simulink model "TRN"  (R2022a)
settings: Solver=FixedStepAuto  StartTime=0.0  StopTime=300  FixedStep=0.04  RelTol=1e-3
PreLoadFcn:
  | load('BusStructureTRNsensor.mat');
  | addpath('C:/MAP');
InitFcn:
  | %load TRNDataBusPILS.mat
  | %addpath(genpath(cd))
  | 
  | load('TPF_WHOLESIM_INPUT_SCENARIOS_AGCAS_N35_10E127_70.mat');
  | 
  | % Add DataBus Path
  | addpath(',,/');
  | addpath('../MAP/');
  | addpath('../MAP/MAP_DB');
  | addpath('../MAP/DVOF');
  | addpath(genpath(cd));
  | load('BusStructureTRN.mat');
undefined symbols (not defined in the file or in its folder): Altitude_INS, INSDataNotValid, Latitude_INS, Longitude_INS, TRN, TRNlib
libraries: simulink_extras x26, aerolibconvert2 x14, sharedtransform x3, dspstat3 x2
(part 1 of 3)
settings Model: Creator=HSU  LastModifiedBy=20225
settings OptimizationCC: DefaultParameterBehavior=Inlined  UseDivisionForNetSlopeComputation=on  GainParamInheritBuiltInType=on  UseFloatMulNetSlope=on  PassReuseOutputArgsAs=Individual arguments  ZeroExternalMemoryAtStartup=off  ZeroInternalMemoryAtStartup=off  OptimizeBlockOrder=speed  DifferentSizesBufferReuse=on  EfficientTunableParamExpr=on
settings DebuggingCC: ParameterTunabilityLossMsg=error  UnconnectedInputMsg=warning  UnconnectedOutputMsg=warning  UnconnectedLineMsg=warning  SFUnexpectedBacktrackingDiag=warning  SFNoUnconditionalDefaultTransitionDiag=warning
settings HardwareCC: ProdBitPerPointer=32  ProdBitPerSizeT=32  ProdBitPerPtrDiffT=32  ProdLargestAtomicInteger=Long  ProdLargestAtomicFloat=Double  ProdEndianess=BigEndian  ProdWordSize=32  ProdHWDeviceType=Freescale->MPC83xx
settings ModelReferenceCC: ModelReferenceNumInstancesAllowed=Single
settings SFSimCC: SimUserLibraries=MAPd.lib WS2_32.LIB  MATLABDynamicMemAlloc=off
settings SFSimCC: SimCustomHeaderCode=|
  | #include "MAP.h"
  | #include "MAPDATA.h"
  | #include "DVOF.h"
  | #include "userDefined.h"
settings SFSimCC: SimUserSources=|
  | MAP.c
  | DVOF.c
  | userDefined.c
settings RTWCC: SystemTargetFile=ert.tlc  GenCodeOnly=on  TemplateMakefile=ert_default_tmf  GenerateReport=on  RTWUseSimCustomCode=on  CustomLibrary=MAPd.lib WS2_32.LIB  BuildConfiguration=Faster Runs  LaunchReport=on  DLArmComputeVersion=19.05
settings RTWCC: CustomHeaderCode=|
  | #include "MAP.h"
  | #include "MAPDATA.h"
  | #include "DVOF.h"
  | #include "userDefined.h"
settings RTWCC: CustomSource=|
  | MAP.c
  | DVOF.c
  | userDefined.c
settings CodeAppCC: ForceParamTrailComments=on  IgnoreCustomStorageClasses=off  OperatorAnnotations=on  SimulinkDataObjDesc=on  SFDataObjDesc=on  MATLABFcnDesc=on  InsertBlockDesc=on  StateflowObjectComments=on  MATLABSourceComments=on  EnableCustomComments=on  ReqsInCode=on
settings ERTTargetCC: TargetLangStandard=C99 (ISO)  UtilityFuncGeneration=Shared location  GenerateSampleERTMain=on  SuppressErrorStatus=on  SupportAbsoluteTime=off  SupportNonFinite=off  SupportComplex=off  ParenthesesLevel=Standards  CastingMode=Standards  InlinedParameterPlacement=NonHierarchical  ERTCustomFileTemplate=example_file_process.tlc  PreserveIfCondition=on  ConvertIfToSwitch=off  EnableSignedLeftShifts=off  EnableSignedRightShifts=off

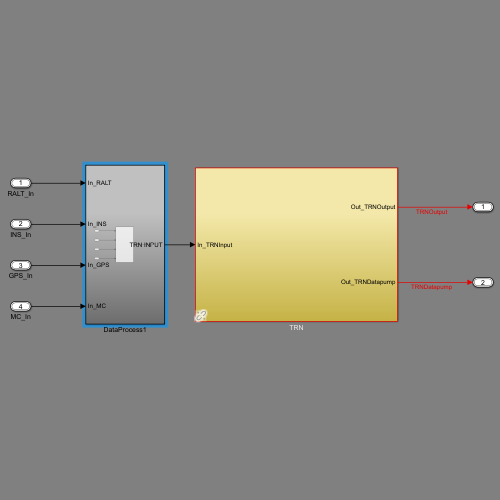
[thumbnail: Simulink's stored preview of the top-level diagram]
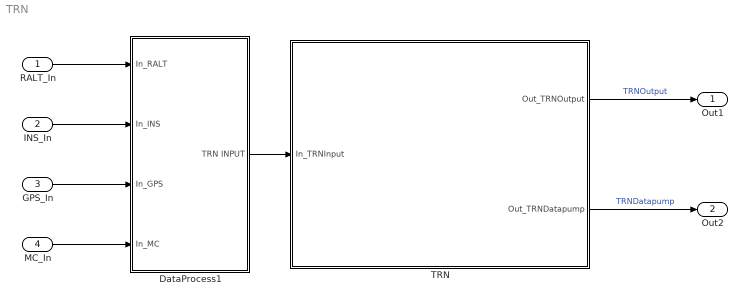
== system TRN ==
  RALT_In : Inport  OutDataTypeStr=Bus: BUS_SENSOR_RALT
  INS_In : Inport  Port=2  OutDataTypeStr=Bus: BUS_SENSOR_INS
  GPS_In : Inport  Port=3  OutDataTypeStr=Bus: BUS_SENSOR_GPS
  MC_In : Inport  Port=4  OutDataTypeStr=Bus: TRN_MC
  DataProcess1 : Subsystem
  TRN : Subsystem  AncestorBlock=TRNlib/TRN
  Out1 : Outport  OutDataTypeStr=Bus: TRNOutput  VectorParamsAs1DForOutWhenUnconnected=off
  Out2 : Outport  Port=2  OutDataTypeStr=Bus: TRNDatapump  VectorParamsAs1DForOutWhenUnconnected=off
  wires:
  TRN/2(Out_TRNDatapump) -> Out2/1  "TRNDatapump"
  TRN/1(Out_TRNOutput) -> Out1/1  "TRNOutput"
  RALT_In/1 -> DataProcess1/1(In_RALT)
  INS_In/1 -> DataProcess1/2(In_INS)
  GPS_In/1 -> DataProcess1/3(In_GPS)
  DataProcess1/1(TRN INPUT) -> TRN/1(In_TRNInput)
  MC_In/1 -> DataProcess1/4(In_MC)

== system TRN/DataProcess1 ==
  In_RALT : Inport
  In_INS : Inport  Port=2
  In_GPS : Inport  Port=3
  In_MC : Inport  Port=4
  Subsystem3 : Subsystem
  TRN INPUT : Outport
  wires:
  In_GPS/1 -> Subsystem3/3(In_GPS)
  In_MC/1 -> Subsystem3/4(In_MC)
  Subsystem3/1(TRN INPUT) -> TRN INPUT/1
  In_RALT/1 -> Subsystem3/1(In_RALT)
  In_INS/1 -> Subsystem3/2(In_INS)

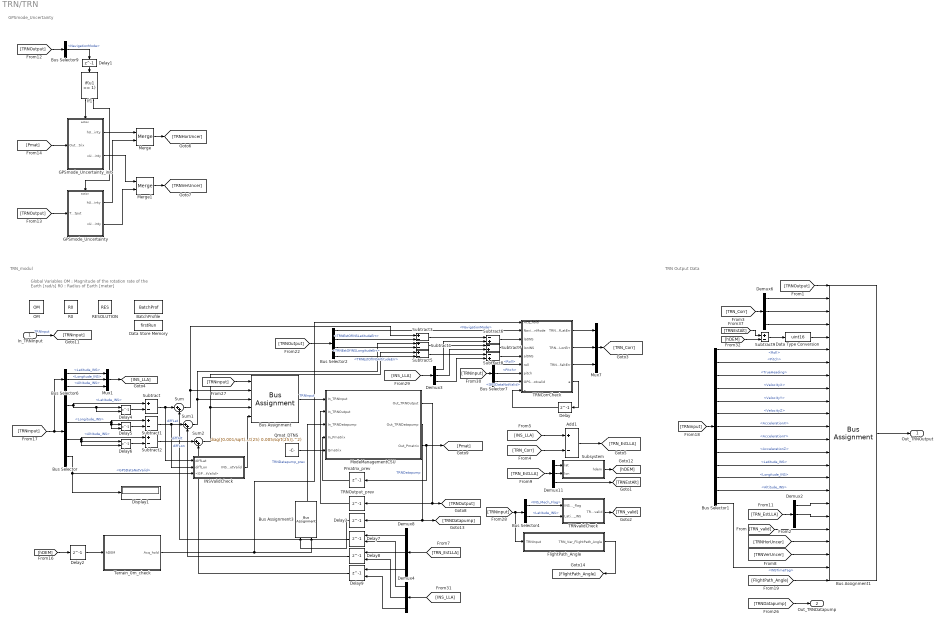
== system TRN/TRN ==
  note: Global Variables
      | OM : Magnitude of the rotation rate of the Earth [rad/s]
      | R0 : Radius of Earth [meter]
  note: GPSmode_Uncertainty
  note: TRN Output Data
  note: TRN_modul
  In_TRNInput : Inport  OutDataTypeStr=Bus: TRNInput
  Add1 : Sum  Inputs=+-
  BatchProfile : DataStoreMemory  DataStoreName=BatchProf  ReadBeforeWriteMsg=warning  WriteAfterWriteMsg=warning  WriteAfterReadMsg=warning  ShowAdditionalParam=off  OutDataTypeStr=double  Dimensions=84200
  Bus Assignment : BusAssignment  AssignedSignals=Latitude_INS,Longitude_INS,Altitude_INS,INSDataNotValid
  Bus Assignment1 : BusAssignment  AssignedSignals=TRNEstOfINSLatitudeErr,TRNEstOfINSLongitudeErr,TRNEstOfINSAltitudeErr,TRNEstHeightAGL,TRN_Roll,TRN_Pitch,TRN_Yaw,TRN_VelocityX,TRN_VelocityY,TRN_VelocityZ,TRN_AccelerationX,TRN_AccelerationY,TRN_AccelerationZ,Latitude_INS,Longitude_INS,Altitude_INS,TRNEstOfLatitude,TRNEstOfLongitude,TRN_valid,TRNHorUncertainty,TRNVerticalUncertainty,TRNTimeTag,TRN_Ver_FlightPath_Angle
  Bus Assignment3 : BusAssignment  AssignedSignals=Acq_hold
  Bus Selector : BusSelector  OutputSignals=Latitude_INS,Longitude_INS,Altitude_INS,GPSDataNotValid
  Bus Selector1 : BusSelector  OutputSignals=Roll,Pitch,TrueHeading,VelocityX,VelocityY,VelocityZ,AccelerationX,AccelerationY,AccelerationZ,Latitude_INS,Longitude_INS,Altitude_INS,INSTimeTag
  Bus Selector2 : BusSelector  OutputSignals=NavigationMode,TRNEstOfINSLatitudeErr,TRNEstOfINSLongitudeErr,TRNEstOfINSAltitudeErr
  Bus Selector4 : BusSelector  OutputSignals=INS_Mech_Flag,Latitude_INS
  Bus Selector6 : BusSelector  OutputSignals=Latitude_INS,Longitude_INS,Altitude_INS
  Bus Selector7 : BusSelector  OutputSignals=Roll,Pitch,GPSDataNotValid
  Bus Selector9 : BusSelector  OutputSignals=NavigationMode
  Data Store Memory : DataStoreMemory  DataStoreName=firstRun  ReadBeforeWriteMsg=warning  WriteAfterWriteMsg=warning  WriteAfterReadMsg=warning  InitialValue=logical(1)  VectorParams1D=off  ShowAdditionalParam=off  OutDataTypeStr=boolean
      settings: LockScale=on
  Data Type Conversion : DataTypeConversion  OutDataTypeStr=uint16  RndMeth=Nearest  SaturateOnIntegerOverflow=off
  Delay : Delay  DelayLength=1
  Delay1 : Delay  DelayLength=1  InitialCondition=1
  Delay2 : Delay  DelayLength=1
  Delay3 : Delay  DelayLength=1  InitialCondition=0
  Delay4 : Delay  DelayLength=1  InitialConditionSource=Input port  InitialCondition=35.2*pi/180
      settings: InputPortMap=u0,p4
  Delay5 : Delay  DelayLength=1  InitialConditionSource=Input port  InitialCondition=35.2*pi/180
      settings: InputPortMap=u0,p4
  Delay6 : Delay  DelayLength=1  InitialConditionSource=Input port  InitialCondition=35.2*pi/180
      settings: InputPortMap=u0,p4
  Delay7 : Delay  DelayLength=1  InitialConditionSource=Input port  InitialCondition=0
      settings: InputPortMap=u0,p4
  Delay8 : Delay  DelayLength=1  InitialConditionSource=Input port  InitialCondition=0
      settings: InputPortMap=u0,p4
  Delay9 : Delay  DelayLength=1  InitialConditionSource=Input port  InitialCondition=0
      settings: InputPortMap=u0,p4
  Demux{2..4,6,8,11} (6 alike) : Demux  Outputs=3
  Display1 : Display
  FlightPath_Angle : Subsystem  TreatAsAtomicUnit=on
  GPSmode_Uncertainty : Subsystem  TreatAsAtomicUnit=on
  GPSmode_Uncertainty_init : Subsystem  TreatAsAtomicUnit=on
  INSValidCheck : Subsystem
  If1 : If  IfExpression=u1 == 1
  Merge : Merge
  Merge1 : Merge
  ModeManagementCSU : Stateflow chart  TreatAsAtomicUnit=on
  Mux1 : Mux  Inputs=3
  Mux7 : Mux  Inputs=3
  OM : DataStoreMemory  DataStoreName=OM  ReadBeforeWriteMsg=warning  WriteAfterWriteMsg=warning  WriteAfterReadMsg=warning  InitialValue=7.27e-5  ShowAdditionalParam=off
  Pmatrix_prev : Delay  DelayLength=1  InitialCondition="diag([0 0 0 0 0 0  10/6378000 10/6378000 13.3 0.0 0.0 0.0 0.00014 0.00014 0.00014 ].^2);"
  Qmat_DTNS : Constant  Value=diag([0.001/sqrt(25) 0.001/sqrt(25) 0.001/sqrt(25) 0.005/sqrt(25) 0.005/sqrt(25) 0.005/sqrt(25)].^2)
  R0 : DataStoreMemory  DataStoreName=R0  ReadBeforeWriteMsg=warning  WriteAfterWriteMsg=warning  WriteAfterReadMsg=warning  InitialValue=6378000  ShowAdditionalParam=off
  RESOLUTION : DataStoreMemory  DataStoreName=RES  ReadBeforeWriteMsg=warning  WriteAfterWriteMsg=warning  WriteAfterReadMsg=warning  InitialValue=3 * 0.000277777777777777 * 0.0174532925199433  ShowAdditionalParam=off  OutDataTypeStr=double
  Subsystem : Subsystem
  Subtract{,1..5,9} (7 alike) : Sum  Inputs=+-
  Subtract6 : Sum  Inputs=-+
  Subtract7 : Sum  Inputs=-+
  Subtract8 : Sum  Inputs=-+
  Sum : Sum  Inputs=|++
  Sum1 : Sum  Inputs=|++
  Sum2 : Sum  Inputs=|++
  TRNCorrCheck : MATLAB Function  TreatAsAtomicUnit=on
  TRNOutput_prev : Delay  DelayLength=1  InitialCondition=struct('NavigationMode', false);
  TRNvalidCheck : MATLAB Function  TreatAsAtomicUnit=on
  Terrain_0m_check : MATLAB Function  TreatAsAtomicUnit=on
  Out_TRNOutput : Outport  OutDataTypeStr=Bus: TRNOutput  VectorParamsAs1DForOutWhenUnconnected=off
  Out_TRNDatapump : Outport  Port=2  OutDataTypeStr=Bus: TRNDatapump  VectorParamsAs1DForOutWhenUnconnected=off
  wires:
  Bus Selector2/3 -> Subtract4/2  "<TRNEstOfINSLongitudeErr>"
  Bus Selector2/2 -> Subtract3/2  "<TRNEstOfINSLatitudeErr>"
  Subsystem/1(hdem) -> [hDEM]
  Bus Selector4/1 -> TRNvalidCheck/1(INS_Mech_flag)  "<INS_Mech_Flag>"
  Bus Selector4/2 -> TRNvalidCheck/2(Latitude_INS)  "<Latitude_INS>"
  [TRN_valid] -> Bus Assignment1/20
  TRNvalidCheck/1(TRN_valid) -> [TRN_valid]
  Bus Assignment/1 -> ModeManagementCSU/1(In_TRNInput)  "TRNInput"
  Bus Selector/2 -> Subtract1/1, Delay5/1, Delay5/2  "<Longitude_INS>"
  Bus Selector1/3 -> Bus Assignment1/8  "<TrueHeading>"
  Bus Selector1/12 -> Bus Assignment1/17  "<Altitude_INS>"
  Bus Selector1/11 -> Bus Assignment1/16  "<Longitude_INS>"
  Bus Selector1/10 -> Bus Assignment1/15  "<Latitude_INS>"
  Bus Selector1/9 -> Bus Assignment1/14  "<AccelerationZ>"
  Bus Selector1/8 -> Bus Assignment1/13  "<AccelerationY>"
  Bus Selector1/7 -> Bus Assignment1/12  "<AccelerationX>"
  Bus Selector1/6 -> Bus Assignment1/11  "<VelocityZ>"
  Bus Selector1/5 -> Bus Assignment1/10  "<VelocityY>"
  Bus Selector1/4 -> Bus Assignment1/9  "<VelocityX>"
  Bus Selector1/2 -> Bus Assignment1/7  "<Pitch>"
  Bus Selector1/1 -> Bus Assignment1/6  "<Roll>"
  In_TRNInput/1 -> [TRNinput]  "TRNInput"
  ModeManagementCSU/1(Out_TRNOutput) -> TRNOutput_prev/1, [TRNOutput]
  ModeManagementCSU/2(Out_TRNDatapump) -> Delay3/1, [TRNDatapump]  "TRNDatapump"
  Pmatrix_prev/1 -> ModeManagementCSU/4(In_Pmatrix)
  TRNOutput_prev/1 -> ModeManagementCSU/2(In_TRNOutput)
  Delay3/1 -> Bus Assignment3/1
  Bus Selector/3 -> Subtract2/1, Delay6/2, Delay6/1  "<Altitude_INS>"
  Bus Selector/1 -> Subtract/1, Delay4/1, Delay4/2  "<Latitude_INS>"
  Delay4/1 -> Subtract/2
  Delay5/1 -> Subtract1/2
  Delay6/1 -> Subtract2/2
  Sum/1 -> Subtract3/1, Bus Assignment/2
  Sum1/1 -> Subtract4/1, Bus Assignment/3
  Sum2/1 -> Subtract5/1, Bus Assignment/4
  Subtract/1 -> Sum/1, INSValidCheck/1(diffLat)  "diffLat"
  Subtract1/1 -> INSValidCheck/2(diffLon), Sum1/1  "diffLon"
  Subtract4/1 -> Subtract7/1
  Subtract2/1 -> Sum2/1  "diffAlt"
  Delay7/1 -> Sum/2
  Delay8/1 -> Sum1/2
  Delay9/1 -> Sum2/2
  Bus Assignment1/1 -> Out_TRNOutput/1
  Subtract9/1 -> Data Type Conversion/1
  Data Type Conversion/1 -> Bus Assignment1/5
  Subtract6/1 -> TRNCorrCheck/3(latINS)
  Subtract7/1 -> TRNCorrCheck/4(lonINS)
  Subtract8/1 -> TRNCorrCheck/5(altINS)
  TRNCorrCheck/3(TRNEstOfaltErr) -> Mux7/3
  [TRN_Corr] -> Demux6/1
  Demux6/1 -> Bus Assignment1/2
  Demux6/2 -> Bus Assignment1/3
  Demux6/3 -> Bus Assignment1/4
  TRNCorrCheck/1(TRNEstOfLatErr) -> Mux7/1
  TRNCorrCheck/2(TRNEstOfLonErr) -> Mux7/2
  Subtract5/1 -> Subtract8/1
  Subtract3/1 -> Subtract6/1
  [TRN_EstLLA] -> Demux8/1
  Demux8/1 -> Delay7/1
  Demux8/2 -> Delay8/1
  Demux8/3 -> Delay9/1
  Mux1/1 -> [INS_LLA]
  Bus Selector6/2 -> Mux1/2  "<Longitude_INS>"
  Bus Selector6/3 -> Mux1/3  "<Altitude_INS>"
  [INS_LLA] -> Add1/1
  [TRN_Corr] -> Add1/2
  Add1/1 -> [TRN_EstLLA]
  Demux11/1 -> Subsystem/1(lat)
  Demux11/2 -> Subsystem/2(lon)
  TRNCorrCheck/4(a) -> Delay/1
  Delay/1 -> TRNCorrCheck/9("a ")
  [TRN_EstLLA] -> Demux11/1
  Qmat_DTNS/1 -> ModeManagementCSU/5(Qmatrix)
  ModeManagementCSU/3(Out_Pmatrix) -> Pmatrix_prev/1, [Pmat]
  INSValidCheck/1(INSDataNotValid) -> Bus Assignment/5
  Bus Selector/4 -> Display1/1, INSValidCheck/3(<GPSDataNotValid>)  "<GPSDataNotValid>"
  Mux7/1 -> [TRN_Corr]
  If1/1 -> GPSmode_Uncertainty_init/Action
  If1/2 -> GPSmode_Uncertainty/Action
  GPSmode_Uncertainty_init/1(hUncertainty) -> Merge/1
  GPSmode_Uncertainty/1(hUncertainty) -> Merge/2
  GPSmode_Uncertainty_init/2(vUncertainty) -> Merge1/1
  GPSmode_Uncertainty/2(vUncertainty) -> Merge1/2
  Bus Selector9/1 -> Delay1/1  "<NavigationMode>"
  Merge/1 -> [TRNHorUncer]
  Merge1/1 -> [TRNVerUncer]
  [TRNHorUncer] -> Bus Assignment1/21
  [TRNVerUncer] -> Bus Assignment1/22
  Demux2/1 -> Bus Assignment1/18
  Demux2/2 -> Bus Assignment1/19
  [TRN_EstLLA] -> Demux2/1
  [TRNOutput] -> Bus Selector9/1
  [TRNOutput] -> GPSmode_Uncertainty/1(TRNOutput)
  [Pmat] -> GPSmode_Uncertainty_init/1(Out_Pmatrix)
  [TRNinput] -> Bus Selector6/1, Bus Selector/1
  [TRNinput] -> Bus Selector1/1
  [TRNDatapump] -> Out_TRNDatapump/1
  [TRNinput] -> Bus Assignment/1
  Delay1/1 -> If1/1
  [TRNOutput] -> Bus Assignment1/1
  Bus Selector2/4 -> Subtract5/2  "<TRNEstOfINSAltitudeErr>"
  [TRNOutput] -> Bus Selector2/1
  [INS_LLA] -> Demux3/1
  Demux3/1 -> Subtract6/2
  Demux3/2 -> Subtract7/2
  Demux3/3 -> Subtract8/2
  [TRNinput] -> Bus Selector7/1
  Bus Selector7/1 -> TRNCorrCheck/6(roll)  "<Roll>"
  Bus Selector7/2 -> TRNCorrCheck/7(pitch)  "<Pitch>"
  Bus Selector6/1 -> Mux1/1  "<Latitude_INS>"
  [INS_LLA] -> Demux4/1
  Demux4/1 -> Delay7/2
  Demux4/2 -> Delay8/2
  Demux4/3 -> Delay9/2
  Bus Selector7/3 -> TRNCorrCheck/8(GPSDataNotvalid)  "<GPSDataNotValid>"
  [hDEM] -> Subtract9/2
  Demux11/3 -> [TRNEstAlt]
  [TRNEstAlt] -> Subtract9/1
  Bus Selector1/13 -> Bus Assignment1/23  "<INSTimeTag>"
  [hDEM] -> Delay2/1
  Delay2/1 -> Terrain_0m_check/1(hDEM)
  Bus Assignment3/1 -> ModeManagementCSU/3(In_TRNDatapump)  "TRNDatapump_prev"
  [TRNinput] -> Bus Selector4/1, FlightPath_Angle/1(TRNInput)
  FlightPath_Angle/1(TRN_Ver_FlightPath_Angle) -> [FlightPath_Angle]
  [FlightPath_Angle] -> Bus Assignment1/24
  Bus Selector2/1 -> TRNCorrCheck/2(NavigationMode)  "<NavigationMode>"
  Terrain_0m_check/1(Acq_hold) -> TRNCorrCheck/1(Acq_hold), Bus Assignment3/2

== system TRN/DataProcess1/Subsystem3 ==
  In_RALT : Inport
  In_INS : Inport  Port=2
  In_GPS : Inport  Port=3
  In_MC : Inport  Port=4
  Bus Creator4 : BusCreator  Inputs=1  OutDataTypeStr=Bus: TRN_MC
  Bus Selector8 : BusSelector  OutputSignals=WeightOnWheels
  Data Type Conversion44 : DataTypeConversion  OutDataTypeStr=boolean  SaturateOnIntegerOverflow=off  RndMeth=Floor
  Dataprocess : Subsystem
  Subsystem : Subsystem
  Subsystem2 : Subsystem
  Subsystem4 : Subsystem
  TRN INPUT : Outport
  wires:
  Data Type Conversion44/1 -> Bus Creator4/1  "WeightOnWheels"
  Subsystem2/1(INS_data) -> Dataprocess/2(In_INS)
  Bus Creator4/1 -> Dataprocess/4(IN_MC)  "MC"
  Subsystem/1(GPS_data) -> Dataprocess/1(In_GPS)
  Dataprocess/1(TRN INPUT) -> TRN INPUT/1
  In_MC/1 -> Bus Selector8/1
  In_GPS/1 -> Subsystem/1(In_GPS)
  In_INS/1 -> Subsystem2/1(In_INS)
  In_RALT/1 -> Subsystem4/1(In_RALT)
  Subsystem4/1(RALT_data) -> Dataprocess/3(In_RALT)
  Bus Selector8/1 -> Data Type Conversion44/1  "<WeightOnWheels>"

== system TRN/TRN/FlightPath_Angle ==
  TRNInput : Inport
  Bus Selector1 : BusSelector  OutputSignals=VelocityX,VelocityY,VelocityZ,Roll,Pitch,TrueHeading
  Degrees to Radians1 : simulink_extras/Transformations/Degrees to Radians
  Degrees to Radians2 : simulink_extras/Transformations/Degrees to Radians
  Degrees to Radians3 : simulink_extras/Transformations/Degrees to Radians
  FlightPath_Angle : MATLAB Function  TreatAsAtomicUnit=on
  Matrix Multiply1 : Product  Multiplication=Matrix(*)
  Mux : Mux  Inputs=3
  Mux2 : Mux  Inputs=3
  Rotation Angles to Direction Cosine Matrix : sharedtransform/Rotation Angles to Direction Cosine Matrix  rotationOrder=ZYX  aMode=aMode
      settings: SourceProductBaseCode=AE,PW,DR,MT,VE
  Selector : Selector  InputPortWidth=3  IndexOptions=Index vector (dialog)  Indices=[3 2 1]  OutputSizes=1
  Transpose : Math  Operator=transpose  SignedPower=on
  TRN_Ver_FlightPath_Angle : Outport
  wires:
  Rotation Angles to Direction Cosine Matrix/1 -> Transpose/1
  Mux2/1 -> Matrix Multiply1/2
  Transpose/1 -> Matrix Multiply1/1
  Matrix Multiply1/1 -> FlightPath_Angle/1(vNED)
  Degrees to Radians1/1 -> Mux/1
  Bus Selector1/5 -> Degrees to Radians2/1  "<Pitch>"
  Mux/1 -> Selector/1
  Degrees to Radians3/1 -> Mux/3
  Degrees to Radians2/1 -> Mux/2
  Bus Selector1/6 -> Degrees to Radians3/1  "<TrueHeading>"
  TRNInput/1 -> Bus Selector1/1
  Bus Selector1/2 -> Mux2/2  "<VelocityY>"
  Bus Selector1/4 -> Degrees to Radians1/1  "<Roll>"
  Bus Selector1/1 -> Mux2/1  "<VelocityX>"
  Bus Selector1/3 -> Mux2/3  "<VelocityZ>"
  Selector/1 -> Rotation Angles to Direction Cosine Matrix/1
  FlightPath_Angle/1(TRN_Ver_FlightPath_Angle) -> TRN_Ver_FlightPath_Angle/1

== system TRN/TRN/GPSmode_Uncertainty ==
  TRNOutput : Inport
  Action Port : ActionPort  ActionPortLabel=else
  Bus Selector : BusSelector  OutputSignals=TRNHorUncertainty,TRNVerticalUncertainty
  Scope : Scope  NumInputPorts=2
  hUncertainty : Outport
  vUncertainty : Outport  Port=2
  wires:
  TRNOutput/1 -> Bus Selector/1
  Bus Selector/1 -> Scope/1, hUncertainty/1  "<TRNHorUncertainty>"
  Bus Selector/2 -> vUncertainty/1, Scope/2  "<TRNVerticalUncertainty>"

== system TRN/TRN/GPSmode_Uncertainty_init ==
  Out_Pmatrix : Inport
  Action Port : ActionPort  ActionPortLabel=if(u1 == 1)
  Uncertainty_init : MATLAB Function  TreatAsAtomicUnit=on
  hUncertainty : Outport
  vUncertainty : Outport  Port=2
  wires:
  Out_Pmatrix/1 -> Uncertainty_init/1(P)
  Uncertainty_init/1(hUncertainty) -> hUncertainty/1
  Uncertainty_init/2(vUncertainty) -> vUncertainty/1

== system TRN/TRN/INSValidCheck ==
  diffLat : Inport
  diffLon : Inport  Port=2
  <GPSDataNotValid> : Inport  Port=3
  INSValidCheck : MATLAB Function  TreatAsAtomicUnit=on
  INSDataNotValid : Outport
  wires:
  diffLon/1 -> INSValidCheck/2(diff_Lon)
  INSValidCheck/1(NotValid) -> INSDataNotValid/1  "INSDataNotValid"
  diffLat/1 -> INSValidCheck/1(diff_Lat)
  <GPSDataNotValid>/1 -> INSValidCheck/3(GPSDataNotValid)

== system TRN/TRN/ModeManagementCSU/AcquisitionCSU ==
  In_TRNInput : Inport  OutDataTypeStr=Bus: TRNInput  PortDimensions=1
  In_TRNDatapump : Inport  Port=2  OutDataTypeStr=Bus: TRNDatapump  PortDimensions=1
  f : TriggerPort  TriggerType=function-call  VariantControl=Variant
      settings: CopyFcn=Stateflow.SLINSF.SimulinkMan.removeBlockPreDeleteFcn  PreDeleteFcn=Stateflow.SLINSF.SimulinkMan.unsafePredeleteFcn
  AcquisitionCSU : Subsystem  TreatAsAtomicUnit=on
  MAD : Outport  VectorParamsAs1DForOutWhenUnconnected=off
  profileCnt : Outport  Port=2  VectorParamsAs1DForOutWhenUnconnected=off
  posUpdate : Outport  Port=3  VectorParamsAs1DForOutWhenUnconnected=off
  residual : Outport  Port=4  VectorParamsAs1DForOutWhenUnconnected=off
  wires:
  In_TRNInput/1 -> AcquisitionCSU/1(In_TRNInput)
  In_TRNDatapump/1 -> AcquisitionCSU/2(In_TRNDatapump)
  AcquisitionCSU/1(MAD) -> MAD/1
  AcquisitionCSU/2(profileCnt) -> profileCnt/1
  AcquisitionCSU/3(posUpdate) -> posUpdate/1
  AcquisitionCSU/4(residual) -> residual/1

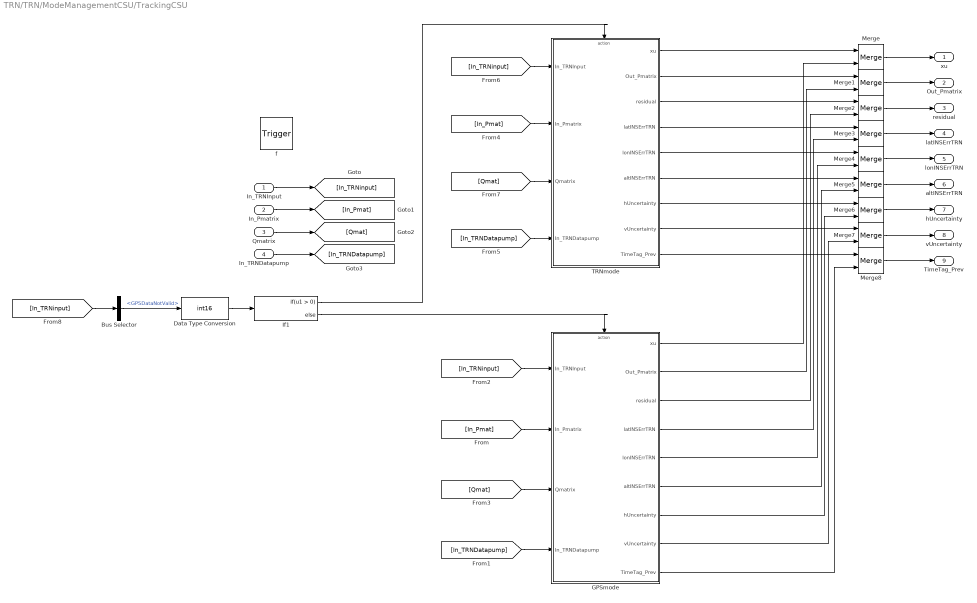
== system TRN/TRN/ModeManagementCSU/TrackingCSU ==
  In_TRNInput : Inport  OutDataTypeStr=Bus: TRNInput  PortDimensions=1
  In_Pmatrix : Inport  Port=2  OutDataTypeStr=double  PortDimensions=[15 15]
  Qmatrix : Inport  Port=3  OutDataTypeStr=double  PortDimensions=[6 6]
  In_TRNDatapump : Inport  Port=4  OutDataTypeStr=Bus: TRNDatapump  PortDimensions=1
  f : TriggerPort  TriggerType=function-call  VariantControl=Variant
      settings: CopyFcn=Stateflow.SLINSF.SimulinkMan.removeBlockPreDeleteFcn  PreDeleteFcn=Stateflow.SLINSF.SimulinkMan.unsafePredeleteFcn
  Bus Selector : BusSelector  OutputSignals=GPSDataNotValid
  Data Type Conversion : DataTypeConversion  OutDataTypeStr=int16  SaturateOnIntegerOverflow=off  RndMeth=Floor
  GPSmode : Subsystem  TreatAsAtomicUnit=on
  If1 : If
  Merge{,1..8} (9 alike) : Merge
  TRNmode : Subsystem  TreatAsAtomicUnit=on
  xu : Outport  VectorParamsAs1DForOutWhenUnconnected=off
  Out_Pmatrix : Outport  Port=2  VectorParamsAs1DForOutWhenUnconnected=off
  residual : Outport  Port=3  VectorParamsAs1DForOutWhenUnconnected=off
  latINSErrTRN : Outport  Port=4  VectorParamsAs1DForOutWhenUnconnected=off
  lonINSErrTRN : Outport  Port=5  VectorParamsAs1DForOutWhenUnconnected=off
  altINSErrTRN : Outport  Port=6  VectorParamsAs1DForOutWhenUnconnected=off
  hUncertainty : Outport  Port=7  VectorParamsAs1DForOutWhenUnconnected=off
  vUncertainty : Outport  Port=8  VectorParamsAs1DForOutWhenUnconnected=off
  TimeTag_Prev : Outport  Port=9  VectorParamsAs1DForOutWhenUnconnected=off
  wires:
  If1/1 -> TRNmode/Action
  If1/2 -> GPSmode/Action
  In_TRNInput/1 -> [In_TRNinput]
  In_Pmatrix/1 -> [In_Pmat]
  Qmatrix/1 -> [Qmat]
  In_TRNDatapump/1 -> [In_TRNDatapump]
  [Qmat] -> GPSmode/3(Qmatrix)
  [In_Pmat] -> GPSmode/2(In_Pmatrix)
  [In_TRNinput] -> GPSmode/1(In_TRNInput)
  [In_TRNDatapump] -> GPSmode/4(In_TRNDatapump)
  [In_TRNDatapump] -> TRNmode/4(In_TRNDatapump)
  [In_TRNinput] -> TRNmode/1(In_TRNInput)
  [In_Pmat] -> TRNmode/2(In_Pmatrix)
  [Qmat] -> TRNmode/3(Qmatrix)
  TRNmode/1(xu) -> Merge/1
  GPSmode/1(xu) -> Merge/2
  TRNmode/2(Out_Pmatrix) -> Merge1/1
  GPSmode/2(Out_Pmatrix) -> Merge1/2
  TRNmode/3(residual) -> Merge2/1
  GPSmode/3(residual) -> Merge2/2
  TRNmode/4(latINSErrTRN) -> Merge3/1
  GPSmode/4(latINSErrTRN) -> Merge3/2
  TRNmode/5(lonINSErrTRN) -> Merge4/1
  GPSmode/5(lonINSErrTRN) -> Merge4/2
  TRNmode/6(altINSErrTRN) -> Merge5/1
  GPSmode/6(altINSErrTRN) -> Merge5/2
  TRNmode/7(hUncertainty) -> Merge6/1
  GPSmode/7(hUncertainty) -> Merge6/2
  TRNmode/8(vUncertainty) -> Merge7/1
  GPSmode/8(vUncertainty) -> Merge7/2
  TRNmode/9(TimeTag_Prev) -> Merge8/1
  GPSmode/9(TimeTag_Prev) -> Merge8/2
  Merge/1 -> xu/1
  Merge1/1 -> Out_Pmatrix/1
  Merge2/1 -> residual/1
  Merge3/1 -> latINSErrTRN/1
  Merge4/1 -> lonINSErrTRN/1
  Merge5/1 -> altINSErrTRN/1
  Merge6/1 -> hUncertainty/1
  Merge7/1 -> vUncertainty/1
  Merge8/1 -> TimeTag_Prev/1
  Bus Selector/1 -> Data Type Conversion/1  "<GPSDataNotValid>"
  Data Type Conversion/1 -> If1/1
  [In_TRNinput] -> Bus Selector/1

== system TRN/TRN/Subsystem ==
  lat : Inport
  lon : Inport  Port=2
  FTGMapCaching : MATLAB Function  TreatAsAtomicUnit=on
  MATLAB Function : MATLAB Function  Commented=on  TreatAsAtomicUnit=on
  hdem : Outport
  wires:
  lat/1 -> FTGMapCaching/1(lat)
  FTGMapCaching/3(hDEM) -> hdem/1
  lon/1 -> FTGMapCaching/2(lon)

== system TRN/DataProcess1/Subsystem3/Dataprocess ==
  In_GPS : Inport
  In_INS : Inport  Port=2
  In_RALT : Inport  Port=3
  IN_MC : Inport  Port=4
  Bus Creator7 : BusCreator  Inputs=42  OutDataTypeStr=Bus: TRNInput
  Bus Selector10 : BusSelector  OutputSignals=WeightOnWheels
  Bus Selector4 : BusSelector  Commented=on  OutputSignals=MAP_hight,Map_Level,Map_size,Map_resolution,bottomLat,leftLon
  Bus Selector5 : BusSelector  OutputSignals=GPSDataNotValid,GPStimeValid,Latitude_GPS,Longitude_GPS,Altitude_GPS,VelocityEast,VelocityNorth,VelocityUp,FigureofMerit,GPSEstHorErr,GPSEstVerticalErr,GPS_State,C_code,P_code
  Bus Selector6 : BusSelector  OutputSignals=INSDataNotValid,INSTimeTag,VelocityX,VelocityY,VelocityZ,Azimuth,Roll,Pitch,TrueHeading,AccelerationX,AccelerationY,AccelerationZ,Latitude_INS,Longitude_INS,Altitude_INS,INS_Alignment_State,INS_Mech_Flag
  Bus Selector7 : BusSelector  OutputSignals=RALTValid,RALTTimeTag,RALTAltitude
  Constant : Constant  Value=0
  Constant13 : Constant  Value=0
  Data Type Conversion : DataTypeConversion  OutDataTypeStr=uint32  SaturateOnIntegerOverflow=off  RndMeth=Floor
  Data Type Conversion11 : DataTypeConversion  OutDataTypeStr=boolean  SaturateOnIntegerOverflow=off  RndMeth=Floor
  TRN INPUT : Outport  OutDataTypeStr=Bus: TRNInput  VectorParamsAs1DForOutWhenUnconnected=off
  wires:
  Bus Selector5/8 -> Bus Creator7/9  "<VelocityUp>"
  Bus Selector6/16 -> Bus Creator7/31  "<INS_Alignment_State>"
  Bus Selector5/7 -> Bus Creator7/8  "<VelocityNorth>"
  In_GPS/1 -> Bus Selector5/1
  Bus Selector5/4 -> Bus Creator7/5  "<Longitude_GPS>"
  Bus Selector5/11 -> Bus Creator7/12  "<GPSEstVerticalErr>"
  Bus Selector5/3 -> Bus Creator7/4  "<Latitude_GPS>"
  Bus Selector6/13 -> Bus Creator7/28  "<Latitude_INS>"
  Bus Selector6/14 -> Bus Creator7/29  "<Longitude_INS>"
  Bus Selector5/12 -> Bus Creator7/13  "<GPS_State>"
  Bus Selector6/9 -> Bus Creator7/24  "<TrueHeading>"
  Bus Selector5/14 -> Bus Creator7/15  "<P_code>"
  Bus Selector6/1 -> Bus Creator7/16  "<INSDataNotValid>"
  Bus Creator7/1 -> TRN INPUT/1
  Data Type Conversion11/1 -> Bus Creator7/1  "SoftResetRequest"
  Bus Selector5/6 -> Bus Creator7/7  "<VelocityEast>"
  Bus Selector6/12 -> Bus Creator7/27  "<AccelerationZ>"
  Bus Selector6/3 -> Bus Creator7/18  "<VelocityX>"
  Bus Selector5/13 -> Bus Creator7/14  "<C_code>"
  Bus Selector6/6 -> Bus Creator7/21  "<Azimuth>"
  Bus Selector5/5 -> Bus Creator7/6  "<Altitude_GPS>"
  Bus Selector6/10 -> Bus Creator7/25  "<AccelerationX>"
  Bus Selector7/3 -> Bus Creator7/35  "<RALTAltitude>"
  In_INS/1 -> Bus Selector6/1
  Bus Selector7/1 -> Bus Creator7/33  "<RALTValid>"
  Bus Selector5/1 -> Bus Creator7/2  "<GPSDataNotValid>"
  Bus Selector10/1 -> Bus Creator7/36  "<WeightOnWheels>"
  Bus Selector6/17 -> Bus Creator7/32  "<INS_Mech_Flag>"
  Bus Selector6/4 -> Bus Creator7/19  "<VelocityY>"
  Bus Selector6/7 -> Bus Creator7/22  "<Roll>"
  Constant13/1 -> Data Type Conversion11/1
  Bus Selector7/2 -> Bus Creator7/34  "<RALTTimeTag>"
  Bus Selector6/5 -> Bus Creator7/20  "<VelocityZ>"
  Bus Selector6/2 -> Bus Creator7/17  "<INSTimeTag>"
  Bus Selector6/8 -> Bus Creator7/23  "<Pitch>"
  Bus Selector5/2 -> Bus Creator7/3  "<GPStimeValid>"
  Bus Selector5/10 -> Bus Creator7/11  "<GPSEstHorErr>"
  Bus Selector6/15 -> Bus Creator7/30  "<Altitude_INS>"
  Bus Selector6/11 -> Bus Creator7/26  "<AccelerationY>"
  Bus Selector5/9 -> Bus Creator7/10  "<FigureofMerit>"
  In_RALT/1 -> Bus Selector7/1
  IN_MC/1 -> Bus Selector10/1
  Constant/1 -> Bus Creator7/39, Bus Creator7/40, Bus Creator7/42, Bus Creator7/41, Bus Creator7/37, Data Type Conversion/1
  Data Type Conversion/1 -> Bus Creator7/38

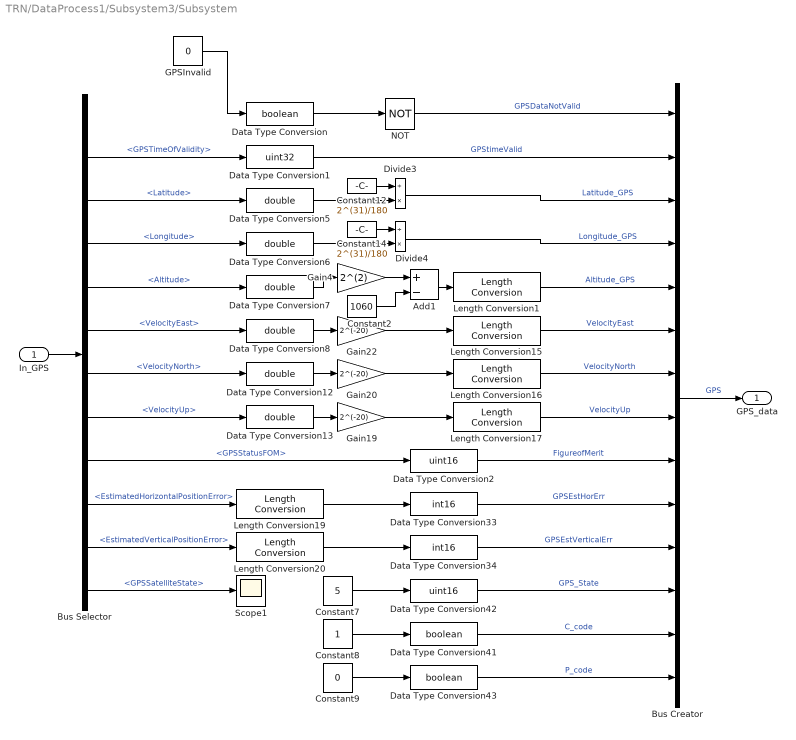
== system TRN/DataProcess1/Subsystem3/Subsystem ==
  In_GPS : Inport
  Add1 : Sum  Inputs=+-
  Bus Creator : BusCreator  Inputs=14  OutDataTypeStr=Bus: TRN_GPS
  Bus Selector : BusSelector  OutputSignals=GPSModeWord,GPSTimeOfValidity,Latitude,Longitude,Altitude,VelocityEast,VelocityNorth,VelocityUp,GPSStatusFOM,EstimatedHorizontalPositionError,EstimatedVerticalPositionError,GPSSatelliteState
  Constant12 : Constant  Value=2^(31)/180
  Constant14 : Constant  Value=2^(31)/180
  Constant2 : Constant  Value=1060
  Constant7 : Constant  Value=5
  Constant8 : Constant
  Constant9 : Constant  Value=0
  Data Type Conversion : DataTypeConversion  OutDataTypeStr=boolean  SaturateOnIntegerOverflow=off  RndMeth=Floor
  Data Type Conversion1 : DataTypeConversion  OutDataTypeStr=uint32  SaturateOnIntegerOverflow=off  RndMeth=Floor
  Data Type Conversion{5..8,12..13} (6 alike) : DataTypeConversion  OutDataTypeStr=double  SaturateOnIntegerOverflow=off  RndMeth=Floor
  Data Type Conversion2 : DataTypeConversion  OutDataTypeStr=uint16  SaturateOnIntegerOverflow=off  RndMeth=Floor
  Data Type Conversion33 : DataTypeConversion  OutDataTypeStr=int16  SaturateOnIntegerOverflow=off  RndMeth=Floor
  Data Type Conversion34 : DataTypeConversion  OutDataTypeStr=int16  SaturateOnIntegerOverflow=off  RndMeth=Floor
  Data Type Conversion41 : DataTypeConversion  OutDataTypeStr=boolean  SaturateOnIntegerOverflow=off  RndMeth=Floor
  Data Type Conversion42 : DataTypeConversion  OutDataTypeStr=uint16  SaturateOnIntegerOverflow=off  RndMeth=Floor
  Data Type Conversion43 : DataTypeConversion  OutDataTypeStr=boolean  SaturateOnIntegerOverflow=off  RndMeth=Floor
  Divide3 : Product  Inputs=/*
  Divide4 : Product  Inputs=/*
  GPSInvalid : Constant  Value=0
  Gain19 : Gain  Gain=2^(-20)
  Gain20 : Gain  Gain=2^(-20)
  Gain22 : Gain  Gain=2^(-20)
  Gain4 : Gain  Gain=2^(2)
  Length Conversion{1,15..17,19..20} (6 alike) : aerolibconvert2/Length Conversion  IU=ft  OU=m
  NOT : Logic  Operator=NOT  IconShape=distinctive  AllPortsSameDT=off  OutDataTypeStr=boolean
  Scope1 : Scope
  GPS_data : Outport
  wires:
  Length Conversion1/1 -> Bus Creator/5  "Altitude_GPS"
  Bus Selector/7 -> Data Type Conversion12/1  "<VelocityNorth>"
  Bus Selector/2 -> Data Type Conversion1/1  "<GPSTimeOfValidity>"
  Bus Selector/3 -> Data Type Conversion5/1  "<Latitude>"
  Gain4/1 -> Add1/1
  Data Type Conversion33/1 -> Bus Creator/10  "GPSEstHorErr"
  Bus Selector/5 -> Data Type Conversion7/1  "<Altitude>"
  Data Type Conversion8/1 -> Gain22/1
  Data Type Conversion41/1 -> Bus Creator/13  "C_code"
  Bus Selector/11 -> Length Conversion20/1  "<EstimatedVerticalPositionError>"
  Gain20/1 -> Length Conversion16/1
  Bus Selector/10 -> Length Conversion19/1  "<EstimatedHorizontalPositionError>"
  Divide3/1 -> Bus Creator/3  "Latitude_GPS"
  Bus Selector/6 -> Data Type Conversion8/1  "<VelocityEast>"
  Data Type Conversion13/1 -> Gain19/1
  Data Type Conversion6/1 -> Divide4/2
  Data Type Conversion34/1 -> Bus Creator/11  "GPSEstVerticalErr"
  Data Type Conversion42/1 -> Bus Creator/12  "GPS_State"
  Gain22/1 -> Length Conversion15/1
  Length Conversion20/1 -> Data Type Conversion34/1
  Data Type Conversion5/1 -> Divide3/2
  Add1/1 -> Length Conversion1/1
  Data Type Conversion1/1 -> Bus Creator/2  "GPStimeValid"
  Gain19/1 -> Length Conversion17/1
  Constant8/1 -> Data Type Conversion41/1
  Data Type Conversion2/1 -> Bus Creator/9  "FigureofMerit"
  Data Type Conversion7/1 -> Gain4/1
  Bus Selector/8 -> Data Type Conversion13/1  "<VelocityUp>"
  Constant7/1 -> Data Type Conversion42/1
  Bus Selector/4 -> Data Type Conversion6/1  "<Longitude>"
  Bus Selector/9 -> Data Type Conversion2/1  "<GPSStatusFOM>"
  Length Conversion17/1 -> Bus Creator/8  "VelocityUp"
  Length Conversion16/1 -> Bus Creator/7  "VelocityNorth"
  Bus Creator/1 -> GPS_data/1  "GPS"
  Data Type Conversion12/1 -> Gain20/1
  Constant2/1 -> Add1/2
  Length Conversion15/1 -> Bus Creator/6  "VelocityEast"
  Length Conversion19/1 -> Data Type Conversion33/1
  Divide4/1 -> Bus Creator/4  "Longitude_GPS"
  Constant9/1 -> Data Type Conversion43/1
  In_GPS/1 -> Bus Selector/1
  Constant14/1 -> Divide4/1
  Constant12/1 -> Divide3/1
  Data Type Conversion43/1 -> Bus Creator/14  "P_code"
  Data Type Conversion/1 -> NOT/1
  NOT/1 -> Bus Creator/1  "GPSDataNotValid"
  Bus Selector/12 -> Scope1/1  "<GPSSatelliteState>"
  GPSInvalid/1 -> Data Type Conversion/1

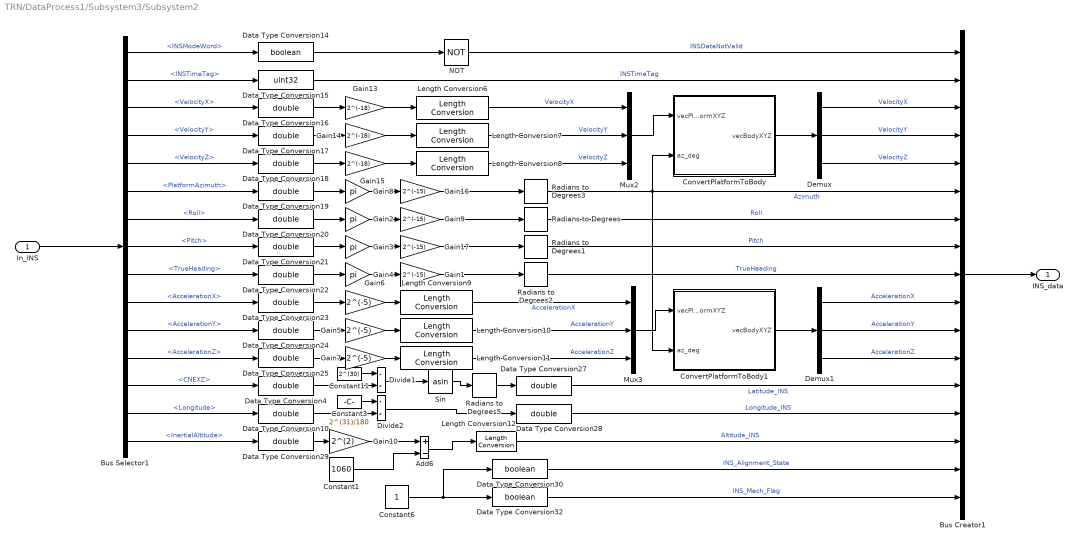
== system TRN/DataProcess1/Subsystem3/Subsystem2 ==
  In_INS : Inport
  Add6 : Sum  Inputs=+-
  Bus Creator1 : BusCreator  Inputs=17  OutDataTypeStr=Bus: TRN_INS
  Bus Selector1 : BusSelector  OutputSignals=INSModeWord,INSTimeTag,VelocityX,VelocityY,VelocityZ,PlatformAzimuth,Roll,Pitch,TrueHeading,AccelerationX,AccelerationY,AccelerationZ,CNEXZ,Longitude,InertialAltitude
  Constant1 : Constant  Value=1060
  Constant11 : Constant  Value=2^(30)
  Constant3 : Constant  Value=2^(31)/180
  Constant6 : Constant
  ConvertPlatformToBody : MATLAB Function  TreatAsAtomicUnit=on
  ConvertPlatformToBody1 : MATLAB Function  TreatAsAtomicUnit=on
  Data Type Conversion{4,10,16..25,27..29} (15 alike) : DataTypeConversion  OutDataTypeStr=double  SaturateOnIntegerOverflow=off  RndMeth=Floor
  Data Type Conversion14 : DataTypeConversion  OutDataTypeStr=boolean  SaturateOnIntegerOverflow=off  RndMeth=Floor
  Data Type Conversion15 : DataTypeConversion  OutDataTypeStr=uint32  SaturateOnIntegerOverflow=off  RndMeth=Floor
  Data Type Conversion30 : DataTypeConversion  OutDataTypeStr=boolean  SaturateOnIntegerOverflow=off  RndMeth=Floor
  Data Type Conversion32 : DataTypeConversion  OutDataTypeStr=boolean  SaturateOnIntegerOverflow=off  RndMeth=Floor
  Demux : Demux  Outputs=3
  Demux1 : Demux  Outputs=3
  Divide1 : Product  Inputs=/*
  Divide2 : Product  Inputs=/*
  Gain{1,9,16..17} (4 alike) : Gain  Gain=2^(-15)
  Gain10 : Gain  Gain=2^(2)
  Gain13 : Gain  Gain=2^(-18)
  Gain14 : Gain  Gain=2^(-18)
  Gain15 : Gain  Gain=2^(-18)
  Gain{2..4,8} (4 alike) : Gain  Gain=pi
  Gain5 : Gain  Gain=2^(-5)
  Gain6 : Gain  Gain=2^(-5)
  Gain7 : Gain  Gain=2^(-5)
  Length Conversion{6..12} (7 alike) : aerolibconvert2/Length Conversion  IU=ft  OU=m
  Mux2 : Mux  Inputs=3
  Mux3 : Mux  Inputs=3
  NOT : Logic  Operator=NOT  IconShape=distinctive  AllPortsSameDT=off  OutDataTypeStr=boolean
  Radians to Degrees{,1..3,5} (5 alike) : simulink_extras/Transformations/Radians to Degrees
  Sin : Trigonometry  Operator=asin
  INS_data : Outport
  wires:
  Length Conversion6/1 -> Mux2/1  "VelocityX"
  Constant6/1 -> Data Type Conversion30/1, Data Type Conversion32/1
  Data Type Conversion32/1 -> Bus Creator1/17  "INS_Mech_Flag"
  Data Type Conversion22/1 -> Gain4/1
  Length Conversion9/1 -> Mux3/1  "AccelerationX"
  Data Type Conversion29/1 -> Gain10/1
  Radians to Degrees2/1 -> Bus Creator1/9  "TrueHeading"
  Data Type Conversion16/1 -> Gain13/1
  Data Type Conversion18/1 -> Gain15/1
  Data Type Conversion15/1 -> Bus Creator1/2  "INSTimeTag"
  Bus Selector1/14 -> Data Type Conversion10/1  "<Longitude>"
  Radians to Degrees5/1 -> Data Type Conversion27/1
  Data Type Conversion24/1 -> Gain5/1
  Sin/1 -> Radians to Degrees5/1
  Constant1/1 -> Add6/2
  Gain14/1 -> Length Conversion7/1
  Data Type Conversion14/1 -> NOT/1
  Bus Selector1/5 -> Data Type Conversion18/1  "<VelocityZ>"
  Data Type Conversion25/1 -> Gain7/1
  Divide2/1 -> Data Type Conversion28/1
  Data Type Conversion19/1 -> Gain8/1
  Bus Selector1/10 -> Data Type Conversion23/1  "<AccelerationX>"
  Data Type Conversion20/1 -> Gain2/1
  Bus Selector1/6 -> Data Type Conversion19/1  "<PlatformAzimuth>"
  Data Type Conversion23/1 -> Gain6/1
  Bus Selector1/7 -> Data Type Conversion20/1  "<Roll>"
  Bus Selector1/2 -> Data Type Conversion15/1  "<INSTimeTag>"
  Bus Selector1/4 -> Data Type Conversion17/1  "<VelocityY>"
  Bus Selector1/3 -> Data Type Conversion16/1  "<VelocityX>"
  Add6/1 -> Length Conversion12/1
  Bus Selector1/15 -> Data Type Conversion29/1  "<InertialAltitude>"
  Bus Selector1/12 -> Data Type Conversion25/1  "<AccelerationZ>"
  Bus Selector1/13 -> Data Type Conversion4/1  "<CNEXZ>"
  Data Type Conversion4/1 -> Divide1/2
  Bus Selector1/9 -> Data Type Conversion22/1  "<TrueHeading>"
  Gain15/1 -> Length Conversion8/1
  Bus Selector1/11 -> Data Type Conversion24/1  "<AccelerationY>"
  Length Conversion12/1 -> Bus Creator1/15  "Altitude_INS"
  Gain6/1 -> Length Conversion9/1
  Data Type Conversion21/1 -> Gain3/1
  Length Conversion8/1 -> Mux2/3  "VelocityZ"
  Data Type Conversion17/1 -> Gain14/1
  Radians to Degrees1/1 -> Bus Creator1/8  "Pitch"
  Length Conversion7/1 -> Mux2/2  "VelocityY"
  Constant3/1 -> Divide2/1
  Gain5/1 -> Length Conversion10/1
  Length Conversion10/1 -> Mux3/2  "AccelerationY"
  Gain7/1 -> Length Conversion11/1
  Radians to Degrees/1 -> Bus Creator1/7  "Roll"
  Divide1/1 -> Sin/1
  Bus Selector1/8 -> Data Type Conversion21/1  "<Pitch>"
  Data Type Conversion10/1 -> Divide2/2
  Data Type Conversion30/1 -> Bus Creator1/16  "INS_Alignment_State"
  Gain10/1 -> Add6/1
  Radians to Degrees3/1 -> ConvertPlatformToBody/2(az_deg), Bus Creator1/6, ConvertPlatformToBody1/2(az_deg)  "Azimuth"
  Length Conversion11/1 -> Mux3/3  "AccelerationZ"
  Constant11/1 -> Divide1/1
  Gain16/1 -> Radians to Degrees3/1
  Gain13/1 -> Length Conversion6/1
  Bus Creator1/1 -> INS_data/1
  In_INS/1 -> Bus Selector1/1
  Gain3/1 -> Gain17/1
  Gain4/1 -> Gain1/1
  Gain2/1 -> Gain9/1
  Gain9/1 -> Radians to Degrees/1
  Gain17/1 -> Radians to Degrees1/1
  Gain1/1 -> Radians to Degrees2/1
  Bus Selector1/1 -> Data Type Conversion14/1  "<INSModeWord>"
  Data Type Conversion27/1 -> Bus Creator1/13  "Latitude_INS"
  Gain8/1 -> Gain16/1
  ConvertPlatformToBody/1(vecBodyXYZ) -> Demux/1
  Demux/1 -> Bus Creator1/3  "VelocityX"
  Demux/2 -> Bus Creator1/4  "VelocityY"
  Demux/3 -> Bus Creator1/5  "VelocityZ"
  Mux2/1 -> ConvertPlatformToBody/1(vecPlatformXYZ)
  Mux3/1 -> ConvertPlatformToBody1/1(vecPlatformXYZ)
  ConvertPlatformToBody1/1(vecBodyXYZ) -> Demux1/1
  Demux1/1 -> Bus Creator1/10  "AccelerationX"
  Demux1/2 -> Bus Creator1/11  "AccelerationY"
  Demux1/3 -> Bus Creator1/12  "AccelerationZ"
  NOT/1 -> Bus Creator1/1  "INSDataNotValid"
  Data Type Conversion28/1 -> Bus Creator1/14  "Longitude_INS"

== system TRN/DataProcess1/Subsystem3/Subsystem4 ==
  In_RALT : Inport
  Add5 : Sum  Inputs=+-
  Bus Creator2 : BusCreator  Inputs=3  OutDataTypeStr=Bus: TRN_RALT
  Bus Selector2 : BusSelector  OutputSignals=RALTModeWord,TimeTag,RadarAltitude
  Constant4 : Constant  Value=50
  Constant5 : Constant  Value=0.625
  Data Type Conversion3 : DataTypeConversion  OutDataTypeStr=double  SaturateOnIntegerOverflow=off  RndMeth=Floor
  Data Type Conversion31 : DataTypeConversion  OutDataTypeStr=uint32  SaturateOnIntegerOverflow=off  RndMeth=Floor
  Data Type Conversion35 : DataTypeConversion  OutDataTypeStr=boolean  SaturateOnIntegerOverflow=off  RndMeth=Floor
  Length Conversion2 : aerolibconvert2/Length Conversion  IU=ft  OU=m
  Product1 : Product
  Scope : Scope  NumInputPorts=2
  RALT_data : Outport
  wires:
  Length Conversion2/1 -> Scope/2, Bus Creator2/3  "RALTAltitude"
  Constant4/1 -> Add5/2
  Bus Creator2/1 -> RALT_data/1  "RALT"
  In_RALT/1 -> Bus Selector2/1
  Data Type Conversion35/1 -> Bus Creator2/1  "RALTValid"
  Add5/1 -> Length Conversion2/1
  Bus Selector2/3 -> Data Type Conversion3/1  "<RadarAltitude>"
  Data Type Conversion3/1 -> Product1/1
  Product1/1 -> Add5/1
  Constant5/1 -> Product1/2
  Data Type Conversion31/1 -> Scope/1, Bus Creator2/2  "RALTTimeTag"
  Bus Selector2/2 -> Data Type Conversion31/1  "<TimeTag>"
  Bus Selector2/1 -> Data Type Conversion35/1  "<RALTModeWord>"

== system TRN/TRN/ModeManagementCSU/AcquisitionCSU/AcquisitionCSU ==
  In_TRNInput : Inport  OutDataTypeStr=Bus: TRNInput
  In_TRNDatapump : Inport  Port=2  OutDataTypeStr=Bus: TRNDatapump
  Bus Selector1 : BusSelector  OutputSignals=profileCnt
  ConvertTRNInput : Subsystem  TreatAsAtomicUnit=on
  CorrelationAnalysis function : MATLAB Function  TreatAsAtomicUnit=on
  Data Store Read : DataStoreRead  DataStoreName=BatchProf  IndexOptions=Index vector (dialog)  Indices=1  OutputSizes=1
  Data Store Write : DataStoreWrite  DataStoreName=BatchProf  IndexOptions=Index vector (dialog)  Indices=1  OutputSizes=1
  Radians to Degrees : simulink_extras/Transformations/Radians to Degrees
  Radians to Degrees1 : simulink_extras/Transformations/Radians to Degrees
  Resolution : Constant  Value=3 * 0.000277777777777777 * 0.0174532925199433
  Scope : Scope  NumInputPorts=4
  Scope1 : Scope
  StoreProfile function : MATLAB Function  TreatAsAtomicUnit=on
  MAD : Outport  VectorParamsAs1DForOutWhenUnconnected=off
  profileCnt : Outport  Port=2  VectorParamsAs1DForOutWhenUnconnected=off
  posUpdate : Outport  Port=3  VectorParamsAs1DForOutWhenUnconnected=off
  residual : Outport  Port=4  VectorParamsAs1DForOutWhenUnconnected=off
  wires:
  ConvertTRNInput/9(flagINS) -> StoreProfile function/11(flagINS)
  CorrelationAnalysis function/8(sum) -> Scope/4
  CorrelationAnalysis function/7(hDEM) -> Scope/3
  CorrelationAnalysis function/5(lonTemp) -> Radians to Degrees1/1
  CorrelationAnalysis function/6(latTemp) -> Radians to Degrees/1
  In_TRNDatapump/1 -> Bus Selector1/1
  In_TRNInput/1 -> ConvertTRNInput/1(TRNInput)
  Bus Selector1/1 -> StoreProfile function/2("profileCnt ")  "<profileCnt>"
  ConvertTRNInput/1(latINS) -> StoreProfile function/3(latINS)
  ConvertTRNInput/2(lonINS) -> StoreProfile function/4(lonINS)
  ConvertTRNInput/3(altINS) -> StoreProfile function/5(altINS)
  ConvertTRNInput/4(altRALT) -> Scope1/1, StoreProfile function/6(RALT)
  Resolution/1 -> CorrelationAnalysis function/3(resolution)
  StoreProfile function/1(batchProfile) -> CorrelationAnalysis function/1("batchProfile ")
  StoreProfile function/2(profileCnt) -> CorrelationAnalysis function/2(profileCnt), profileCnt/1
  CorrelationAnalysis function/2(MAD) -> MAD/1
  CorrelationAnalysis function/1(posUpdate) -> posUpdate/1
  CorrelationAnalysis function/3(residual) -> residual/1
  StoreProfile function/3(gridSize) -> CorrelationAnalysis function/4(gridSize)
  Data Store Read/1 -> StoreProfile function/1("batchProfile ")
  CorrelationAnalysis function/4(batchProfile) -> Data Store Write/1
  ConvertTRNInput/5(latGPS) -> StoreProfile function/7(latGPS)
  ConvertTRNInput/6(lonGPS) -> StoreProfile function/8(lonGPS)
  ConvertTRNInput/7(altGPS) -> StoreProfile function/9(altGPS)
  ConvertTRNInput/8(flagGPS) -> StoreProfile function/10(flagGPS)
  Radians to Degrees/1 -> Scope/1
  Radians to Degrees1/1 -> Scope/2

== system TRN/TRN/ModeManagementCSU/TrackingCSU/GPSmode ==
  In_TRNInput : Inport  OutDataTypeStr=Bus: TRNInput  PortDimensions=1
  In_Pmatrix : Inport  Port=2  OutDataTypeStr=double  PortDimensions=[15 15]
  Qmatrix : Inport  Port=3  OutDataTypeStr=double  PortDimensions=[6 6]
  In_TRNDatapump : Inport  Port=4  OutDataTypeStr=Bus: TRNDatapump  PortDimensions=1
  Action Port : ActionPort  ActionPortLabel=else
  Rmat_DTNS_GPS : Constant  Value=diag([ (6.6/sqrt(25))^2 (6.6/sqrt(25))^2 (1/sqrt(25))^2 (0.5/sqrt(25))^2 (0.5/sqrt(25))^2 (0.5/sqrt(25))^2 ]);
  TrackingCSU_GPS : Subsystem  TreatAsAtomicUnit=on
  xu : Outport  VectorParamsAs1DForOutWhenUnconnected=off
  Out_Pmatrix : Outport  Port=2  VectorParamsAs1DForOutWhenUnconnected=off
  residual : Outport  Port=3  VectorParamsAs1DForOutWhenUnconnected=off
  latINSErrTRN : Outport  Port=4  VectorParamsAs1DForOutWhenUnconnected=off
  lonINSErrTRN : Outport  Port=5  VectorParamsAs1DForOutWhenUnconnected=off
  altINSErrTRN : Outport  Port=6  VectorParamsAs1DForOutWhenUnconnected=off
  hUncertainty : Outport  Port=7  VectorParamsAs1DForOutWhenUnconnected=off
  vUncertainty : Outport  Port=8  VectorParamsAs1DForOutWhenUnconnected=off
  TimeTag_Prev : Outport  Port=9  VectorParamsAs1DForOutWhenUnconnected=off
  wires:
  TrackingCSU_GPS/3(residual) -> residual/1
  TrackingCSU_GPS/9(Timetag_prev) -> TimeTag_Prev/1
  TrackingCSU_GPS/4(latINSErrTRN) -> latINSErrTRN/1
  TrackingCSU_GPS/2(P) -> Out_Pmatrix/1
  TrackingCSU_GPS/5(lonINSErrTRN) -> lonINSErrTRN/1
  Qmatrix/1 -> TrackingCSU_GPS/3(Qmatrix)
  TrackingCSU_GPS/8(vUncertainty) -> vUncertainty/1
  TrackingCSU_GPS/6(altINSErrTRN) -> altINSErrTRN/1
  In_TRNDatapump/1 -> TrackingCSU_GPS/5(In_TRNDatapump)
  In_Pmatrix/1 -> TrackingCSU_GPS/2(Pmatrix)
  TrackingCSU_GPS/1(xu) -> xu/1
  In_TRNInput/1 -> TrackingCSU_GPS/1(In_TRNInput)
  TrackingCSU_GPS/7(hUncertainty) -> hUncertainty/1
  Rmat_DTNS_GPS/1 -> TrackingCSU_GPS/4(Rmatrix)

== system TRN/TRN/ModeManagementCSU/TrackingCSU/TRNmode ==
  In_TRNInput : Inport  OutDataTypeStr=Bus: TRNInput  PortDimensions=1
  In_Pmatrix : Inport  Port=2  OutDataTypeStr=double  PortDimensions=[15 15]
  Qmatrix : Inport  Port=3  OutDataTypeStr=double  PortDimensions=[6 6]
  In_TRNDatapump : Inport  Port=4  OutDataTypeStr=Bus: TRNDatapump  PortDimensions=1
  Action Port : ActionPort  ActionPortLabel=if(u1 > 0)
  Rmat_DTNS_TRN : Constant  Value=diag((35/sqrt(25))^2);
  TrackingCSU_TRN : Subsystem  TreatAsAtomicUnit=on
  xu : Outport  VectorParamsAs1DForOutWhenUnconnected=off
  Out_Pmatrix : Outport  Port=2  VectorParamsAs1DForOutWhenUnconnected=off
  residual : Outport  Port=3  VectorParamsAs1DForOutWhenUnconnected=off
  latINSErrTRN : Outport  Port=4  VectorParamsAs1DForOutWhenUnconnected=off
  lonINSErrTRN : Outport  Port=5  VectorParamsAs1DForOutWhenUnconnected=off
  altINSErrTRN : Outport  Port=6  VectorParamsAs1DForOutWhenUnconnected=off
  hUncertainty : Outport  Port=7  VectorParamsAs1DForOutWhenUnconnected=off
  vUncertainty : Outport  Port=8  VectorParamsAs1DForOutWhenUnconnected=off
  TimeTag_Prev : Outport  Port=9  VectorParamsAs1DForOutWhenUnconnected=off
  wires:
  TrackingCSU_TRN/9(Timetag_prev) -> TimeTag_Prev/1
  TrackingCSU_TRN/4(latINSErrTRN) -> latINSErrTRN/1
  In_TRNInput/1 -> TrackingCSU_TRN/1(In_TRNInput)
  TrackingCSU_TRN/2(P) -> Out_Pmatrix/1
  TrackingCSU_TRN/3(residual) -> residual/1
  TrackingCSU_TRN/7(hUncertainty) -> hUncertainty/1
  TrackingCSU_TRN/6(altINSErrTRN) -> altINSErrTRN/1
  In_Pmatrix/1 -> TrackingCSU_TRN/2(Pmatrix)
  Qmatrix/1 -> TrackingCSU_TRN/3(Qmatrix)
  TrackingCSU_TRN/1(xu) -> xu/1
  TrackingCSU_TRN/5(lonINSErrTRN) -> lonINSErrTRN/1
  Rmat_DTNS_TRN/1 -> TrackingCSU_TRN/4(Rmatrix)
  In_TRNDatapump/1 -> TrackingCSU_TRN/5(In_TRNDatapump)
  TrackingCSU_TRN/8(vUncertainty) -> vUncertainty/1

== system TRN/TRN/ModeManagementCSU/AcquisitionCSU/AcquisitionCSU/ConvertTRNInput ==
  TRNInput : Inport  OutDataTypeStr=Bus: TRNInput
  Bus Selector1 : BusSelector  OutputSignals=Latitude_INS,Longitude_INS,Altitude_INS,RALTAltitude,GPSDataNotValid,Latitude_GPS,Longitude_GPS,Altitude_GPS,INSDataNotValid
  Degrees to Radians{1..2,4..5} (4 alike) : simulink_extras/Transformations/Degrees to Radians
  latINS : Outport  VectorParamsAs1DForOutWhenUnconnected=off
  lonINS : Outport  Port=2  VectorParamsAs1DForOutWhenUnconnected=off
  altINS : Outport  Port=3  VectorParamsAs1DForOutWhenUnconnected=off
  altRALT : Outport  Port=4  VectorParamsAs1DForOutWhenUnconnected=off
  latGPS : Outport  Port=5  VectorParamsAs1DForOutWhenUnconnected=off
  lonGPS : Outport  Port=6  VectorParamsAs1DForOutWhenUnconnected=off
  altGPS : Outport  Port=7  VectorParamsAs1DForOutWhenUnconnected=off
  flagGPS : Outport  Port=8  VectorParamsAs1DForOutWhenUnconnected=off
  flagINS : Outport  Port=9  VectorParamsAs1DForOutWhenUnconnected=off
  wires:
  Bus Selector1/9 -> flagINS/1  "<INSDataNotValid>"
  Bus Selector1/2 -> Degrees to Radians4/1  "<Longitude_INS>"
  Bus Selector1/1 -> Degrees to Radians5/1  "<Latitude_INS>"
  Bus Selector1/4 -> altRALT/1  "<RALTAltitude>"
  Degrees to Radians4/1 -> lonINS/1
  Degrees to Radians5/1 -> latINS/1
  TRNInput/1 -> Bus Selector1/1
  Bus Selector1/3 -> altINS/1  "<Altitude_INS>"
  Bus Selector1/5 -> flagGPS/1  "<GPSDataNotValid>"
  Bus Selector1/6 -> Degrees to Radians1/1  "<Latitude_GPS>"
  Bus Selector1/7 -> Degrees to Radians2/1  "<Longitude_GPS>"
  Bus Selector1/8 -> altGPS/1  "<Altitude_GPS>"
  Degrees to Radians2/1 -> lonGPS/1
  Degrees to Radians1/1 -> latGPS/1
